simulink model "simu1"  (R2019b)
settings: Solver=VariableStepAuto  StartTime=0.0  StopTime=10.0  RelTol=1e-3
settings Model: Creator=Admin  LastModifiedBy=Admin

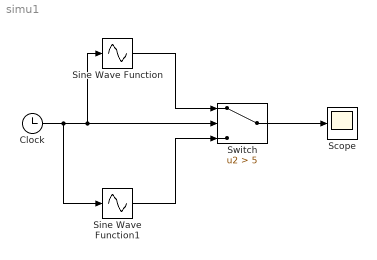
== system simu1 ==
  Clock : Clock
  Scope : Scope
  Sine Wave Function : Sin  TimeSource=Use external signal  Amplitude=5  SampleTime=0
  Sine Wave Function1 : Sin  TimeSource=Use external signal  Amplitude=3  Frequency=2  Phase=0.5  SampleTime=0
  Switch : Switch  Criteria=u2 > Threshold  Threshold=5
  wires:
  Clock/1 -> Sine Wave Function/1, Switch/2, Sine Wave Function1/1
  Sine Wave Function/1 -> Switch/1
  Sine Wave Function1/1 -> Switch/3
  Switch/1 -> Scope/1
